simulink model "full"  (R2020a)
settings: Solver=VariableStepAuto  StartTime=0.0  StopTime=10.0  RelTol=1e-3
libraries: aerolibconvert2 x1
settings Model: Creator=decla  LastModifiedBy=decla

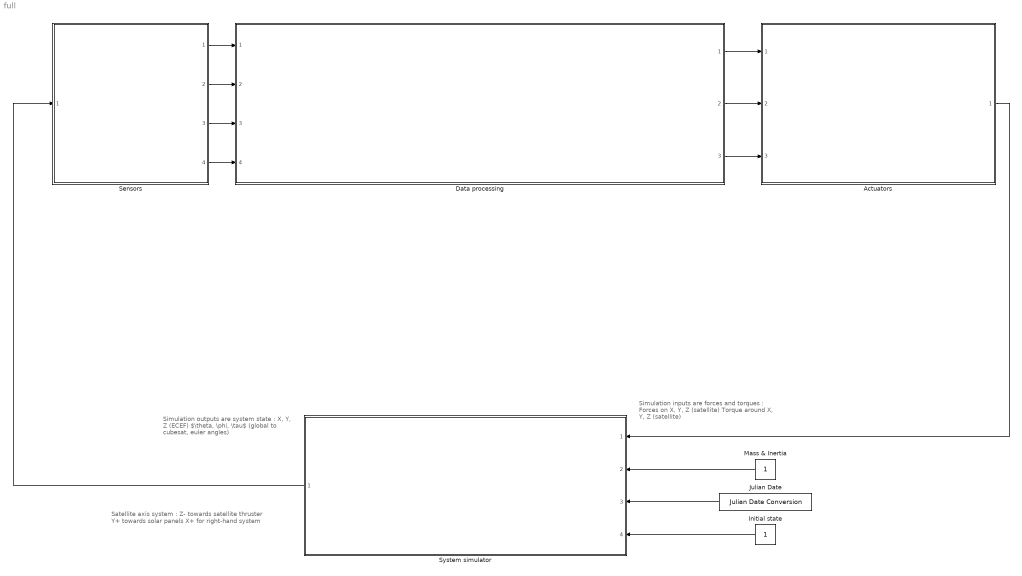
== system full ==
  note: Simulation outputs are system state :
      | X, Y, Z (ECEF)
      | $\theta, \phi, \tau$ (global to cubesat, euler angles)
  note: Simulation inputs are forces and torques :
      | Forces on X, Y, Z (satellite)
      | Torque around X, Y, Z (satellite)
  note: Satellite axis system :
      | Z- towards satellite thruster
      | Y+ towards solar panels
      | X+ for right-hand system
  Actuators : Subsystem  ReferencedSubsystem=Actuators
  Data processing : Subsystem  ReferencedSubsystem=Data_processing
  Initial state : Constant
  Julian Date : aerolibconvert2/Julian Date Conversion  year=2004  month=October  day=10  hour=12  min=21  sec=0  modflag=off  deltaT=None  errorflag=Error
      settings: SourceProductBaseCode=AE
  Mass & Inertia : Constant
  Sensors : Subsystem  ReferencedSubsystem=Sensors
  System simulator : Subsystem  ReferencedSubsystem=Physical_system
  wires:
  Data processing/3 -> Actuators/3
  Actuators/1 -> System simulator/1
  System simulator/1 -> Sensors/1
  Sensors/4 -> Data processing/4
  Sensors/3 -> Data processing/3
  Sensors/2 -> Data processing/2
  Sensors/1 -> Data processing/1
  Data processing/2 -> Actuators/2
  Data processing/1 -> Actuators/1
  Mass & Inertia/1 -> System simulator/2
  Julian Date/1 -> System simulator/3
  Initial state/1 -> System simulator/4
